simulink model "Symmetry_COPY"  (Simulink 8.1)
settings: Solver=ode23t  StartTime=0.0  StopTime=tfin  RelTol=1e-4
values from neighbouring files (symbols this model uses):
  amp_feedback_saturation = 400    [Symmetry_ini_COPY.m]
  Butterworth_filter_order = 8    [Sketch_controller_model_ini.m]    (also in Symmetry_ini.m; Symmetry_ini_COPY.m)
  C_Network = [0, 0, 0]    [Symmetry_ini.m]    (also in Symmetry_ini_COPY.m)
  Capacitive_Load_R_RC = [30e-3,  60e-3,  40e-3;                                1e-3, 5e-3, 3e-3]    [Symmetry_ini.m]    (also in Symmetry_ini_COPY.m = [60e-3,  120e-3,  80e-3;                                1e-3)
  Capacitive_Load_R_Switching_Sequence = Capacitive_Load_R_Switching_Sequence_'    [Symmetry_ini.m]    (also in Symmetry_ini_COPY.m = ones(3,tfin/Capacitive_Load_R_Switching_Speed(1))')
  Capacitive_Load_R_Switching_Speed = [0.01,0.01,0.01]    [Symmetry_ini.m]    (also in Symmetry_ini_COPY.m)
  Capacitive_Load_S_RC = [30e-3,  60e-3,  40e-3;                                1e-3, 5e-3, 3e-3]    [Symmetry_ini.m]    (also in Symmetry_ini_COPY.m = [60e-3,  120e-3,  80e-3;                                1e-3)
  Capacitive_Load_S_Switching_Sequence = Capacitive_Load_S_Switching_Sequence_'    [Symmetry_ini.m]    (also in Symmetry_ini_COPY.m = ones(3,tfin/Capacitive_Load_R_Switching_Speed(1))')
  Capacitive_Load_S_Switching_Speed = [0.01,0.01,0.01]    [Symmetry_ini.m]    (also in Symmetry_ini_COPY.m)
  Capacitive_Load_T_RC = [30e-3,  60e-3,  40e-3;                                1e-3, 5e-3, 3e-3]    [Symmetry_ini.m]    (also in Symmetry_ini_COPY.m = [60e-3,  120e-3,  80e-3;                                1e-3)
  Capacitive_Load_T_Switching_Sequence = Capacitive_Load_T_Switching_Sequence_'    [Symmetry_ini.m]    (also in Symmetry_ini_COPY.m = ones(3,tfin/Capacitive_Load_R_Switching_Speed(1))')
  Capacitive_Load_T_Switching_Speed = [0.01,0.01,0.01]    [Symmetry_ini.m]    (also in Symmetry_ini_COPY.m)
  i = str2num(answer{1})/sample    [Test_intersect.m]
  initial_value = [1,1,1,                  0,-2/3*pi,-4/3*pi]    [Symmetry_ini_COPY.m]
  L_Network = [3.185e-3, 3.185e-3, 3.185e-3, 3.185e-3]    [Symmetry_ini.m]    (also in Symmetry_ini_COPY.m)
  L_Source = [3.185e-3, 3.185e-3, 3.185e-3]    [Sketch_controller_model_ini.m]    (also in Symmetry_ini.m; Symmetry_ini_COPY.m)
  Load_R = [50,50,50]    [Symmetry_ini.m]    (also in Symmetry_ini_COPY.m)
  Load_RL = [35.35,   35.35,   35.35;                  0.1125,  0.1125,  0.1125]    [Symmetry_ini.m]    (also in Symmetry_ini_COPY.m)
  Load_Wire_Resistance = [0.1,0.2]    [Symmetry_ini.m]    (also in Symmetry_ini_COPY.m)
  P_gain = 0.01    [Symmetry_ini_COPY.m]
  phase_feedback_saturation = pi    (= 3.14159265359)    [Symmetry_ini_COPY.m]
  Phase_Source = [0,2/3*pi,4/3*pi]    [Sketch_controller_model_ini.m]    (also in Symmetry_REAL_TIME_ini.m = [0,-2/3*pi,-4/3*pi]; Symmetry_ini.m; Symmetry_ini_COPY.m = [0,-2/3*pi,-4/3*pi])
  R_Network = [0.4, 0.4, 0.4, 0.4]    [Symmetry_ini.m]    (also in Symmetry_ini_COPY.m)
  R_Source = [0.4, 0.4, 0.4]    [Sketch_controller_model_ini.m]    (also in Symmetry_ini.m; Symmetry_ini_COPY.m)
  sample = 10e-5    (= 0.0001)    [Inverter_ini.m]    (also in Sketch_controller_model_ini.m; Symmetry_REAL_TIME_ini.m; Symmetry_ini.m; Symmetry_ini_COPY.m)
  Source_Frequency = [50,50,50]    [Sketch_controller_model_ini.m]    (also in Symmetry_ini.m; Symmetry_ini_COPY.m)
  Start_Control = 0.1    [Symmetry_ini_COPY.m]
  step_size = [5,5,5,                  0.32,0.32,0.32]    [Symmetry_ini_COPY.m]
  Switch_Load_R = [1,1,1]    [Symmetry_ini.m]    (also in Symmetry_ini_COPY.m = [1,0,0])
  Switch_Load_RC = [1,1,1]    [Symmetry_ini.m]    (also in Symmetry_ini_COPY.m = [0,0,1])
  Switch_Load_RL = [1,1,1]    [Symmetry_ini.m]    (also in Symmetry_ini_COPY.m = [0,1,0])
  test_step = [1,1,1,                  0.08,0.08,0.08]    [Symmetry_ini_COPY.m]
  Urms_Source = [230,230,230]    [Sketch_controller_model_ini.m]    (also in Symmetry_REAL_TIME_ini.m; Symmetry_ini.m; Symmetry_ini_COPY.m)
libraries: powerlib x87, simulink x27, powerlib_extras x12, dspsigops x10, commsequence2 x6, dspxfrm3 x3, dsparch4 x3
(part 2 of 2)

== system Symmetry_COPY/Load System/Loads/Inductive_Loads_RST ==
  Breaker1 : powerlib/Elements/Breaker  BreakerResistance=0.01  InitialState=0  SnubberResistance=1e7  SnubberCapacitance=inf  SwitchingTimes="[ 1/60  5/60 ]"  External=on  Measurements=None  MoreParameters=off  NoBreakLoop=off
  Breaker13 : powerlib/Elements/Breaker  BreakerResistance=0.01  InitialState=0  SnubberResistance=1e7  SnubberCapacitance=inf  SwitchingTimes="[ 1/60  5/60 ]"  External=on  Measurements=None  MoreParameters=off  NoBreakLoop=off
  Breaker2 : powerlib/Elements/Breaker  BreakerResistance=0.01  InitialState=0  SnubberResistance=1e7  SnubberCapacitance=inf  SwitchingTimes="[ 1/60  5/60 ]"  External=on  Measurements=None  MoreParameters=off  NoBreakLoop=off
  Constant : Constant  Value=Switch_Load_RL(1)
  Constant1 : Constant  Value=Switch_Load_RL(2)
  Constant2 : Constant  Value=Switch_Load_RL(3)
  RL_load : powerlib/Elements/Series RLC Branch  LConnTagsString=__new0  RConnTagsString=__new0  BranchType=RL  Resistance=Load_RL(1,1)  Inductance=Load_RL(2,1)  SetiL0=off  InitialCurrent=0  Capacitance=1.0  Setx0=off  InitialVoltage=0  Measurements=None
  RL_load1 : powerlib/Elements/Series RLC Branch  LConnTagsString=__new0  RConnTagsString=__new0  BranchType=RL  Resistance=Load_RL(1,2)  Inductance=Load_RL(2,2)  SetiL0=off  InitialCurrent=0  Capacitance=1.0  Setx0=off  InitialVoltage=0  Measurements=None
  RL_load2 : powerlib/Elements/Series RLC Branch  LConnTagsString=__new0  RConnTagsString=__new0  BranchType=RL  Resistance=Load_RL(1,3)  Inductance=Load_RL(2,3)  SetiL0=off  InitialCurrent=0  Capacitance=1.0  Setx0=off  InitialVoltage=0  Measurements=None
  R : PMIOPort  Port=1  Side=Left
  S : PMIOPort  Port=2  Side=Left
  T : PMIOPort  Port=3  Side=Left
  N : PMIOPort  Port=4  Side=Right
  wires:
  Constant/1 -> Breaker13/1
  Constant1/1 -> Breaker1/1
  Constant2/1 -> Breaker2/1
  connections:
  RL_load/RConn1 -- RL_load1/RConn1 -- RL_load2/RConn1 -- N/RConn1
  R/RConn1 -- Breaker13/LConn1
  Breaker1/LConn1 -- S/RConn1
  Breaker2/LConn1 -- T/RConn1
  Breaker13/RConn1 -- RL_load/LConn1
  RL_load1/LConn1 -- Breaker1/RConn1
  RL_load2/LConn1 -- Breaker2/RConn1

== system Symmetry_COPY/Load System/Loads/Ohmic_Loads_RST ==
  Breaker1 : powerlib/Elements/Breaker  BreakerResistance=0.01  InitialState=0  SnubberResistance=1e7  SnubberCapacitance=inf  SwitchingTimes="[ 1/60  5/60 ]"  External=on  Measurements=None  MoreParameters=off  NoBreakLoop=off
  Breaker13 : powerlib/Elements/Breaker  BreakerResistance=0.01  InitialState=0  SnubberResistance=1e7  SnubberCapacitance=inf  SwitchingTimes="[ 1/60  5/60 ]"  External=on  Measurements=None  MoreParameters=off  NoBreakLoop=off
  Breaker2 : powerlib/Elements/Breaker  BreakerResistance=0.01  InitialState=0  SnubberResistance=1e7  SnubberCapacitance=inf  SwitchingTimes="[ 1/60  5/60 ]"  External=on  Measurements=None  MoreParameters=off  NoBreakLoop=off
  Constant : Constant  Value=Switch_Load_R(1)
  Constant1 : Constant  Value=Switch_Load_R(2)
  Constant2 : Constant  Value=Switch_Load_R(3)
  R_load : powerlib/Elements/Series RLC Branch  LConnTagsString=__new0  RConnTagsString=__new0  BranchType=R  Resistance=Load_R(1)  Inductance=0.003185  SetiL0=off  InitialCurrent=0  Capacitance=1.0  Setx0=off  InitialVoltage=0  Measurements=None
  R_load1 : powerlib/Elements/Series RLC Branch  LConnTagsString=__new0  RConnTagsString=__new0  BranchType=R  Resistance=Load_R(2)  Inductance=0.003185  SetiL0=off  InitialCurrent=0  Capacitance=1.0  Setx0=off  InitialVoltage=0  Measurements=None
  R_load2 : powerlib/Elements/Series RLC Branch  LConnTagsString=__new0  RConnTagsString=__new0  BranchType=R  Resistance=Load_R(3)  Inductance=0.003185  SetiL0=off  InitialCurrent=0  Capacitance=1.0  Setx0=off  InitialVoltage=0  Measurements=None
  R : PMIOPort  Port=1  Side=Left
  S : PMIOPort  Port=2  Side=Left
  T : PMIOPort  Port=3  Side=Left
  N : PMIOPort  Port=4  Side=Right
  wires:
  Constant/1 -> Breaker13/1
  Constant1/1 -> Breaker1/1
  Constant2/1 -> Breaker2/1
  connections:
  R_load/RConn1 -- R_load1/RConn1 -- R_load2/RConn1 -- N/RConn1
  Breaker13/LConn1 -- R/RConn1
  Breaker13/RConn1 -- R_load/LConn1
  Breaker1/LConn1 -- S/RConn1
  R_load1/LConn1 -- Breaker1/RConn1
  Breaker2/LConn1 -- T/RConn1
  R_load2/LConn1 -- Breaker2/RConn1

== system Symmetry_COPY/Load System/Log_Signals/3_Phase_P_Q ==
  U_RMS : Inport
  I_RMS : Inport  Port=2
  Demux1 : Demux  Outputs=3
  Demux3 : Demux  Outputs=3
  Mux4 : Mux  Inputs=3
  P Q in3 : powerlib_extras/Measurements/Active & Reactive Power  f1=Source_Frequency(1)
  P Q in4 : powerlib_extras/Measurements/Active & Reactive Power  f1=Source_Frequency(2)
  P Q in5 : powerlib_extras/Measurements/Active & Reactive Power  f1=Source_Frequency(3)
  P_Q_RMS : Outport
  wires:
  I_RMS/1 -> Demux1/1
  Demux1/3 -> P Q in5/2
  Demux1/2 -> P Q in4/2
  Demux1/1 -> P Q in3/2
  Demux3/3 -> P Q in5/1
  Demux3/2 -> P Q in4/1
  Demux3/1 -> P Q in3/1
  P Q in5/1 -> Mux4/3
  Mux4/1 -> P_Q_RMS/1
  U_RMS/1 -> Demux3/1
  P Q in4/1 -> Mux4/2
  P Q in3/1 -> Mux4/1

== system Symmetry_COPY/Load System/Log_Signals/3_Phase_RMS ==
  U_RST : Inport
  Demux5 : Demux  Outputs=3
  Mux2 : Mux  Inputs=3
  RMS1 : powerlib_extras/Measurements/RMS  f1=Source_Frequency(2)
  RMS2 : powerlib_extras/Measurements/RMS  f1=Source_Frequency(3)
  RMS6 : powerlib_extras/Measurements/RMS  f1=Source_Frequency(1)
  U_RMS : Outport
  wires:
  RMS2/1 -> Mux2/3
  Demux5/2 -> RMS1/1
  U_RST/1 -> Demux5/1
  Demux5/3 -> RMS2/1
  RMS6/1 -> Mux2/1
  Demux5/1 -> RMS6/1
  RMS1/1 -> Mux2/2
  Mux2/1 -> U_RMS/1

== system Symmetry_COPY/Load System/Log_Signals/3_Phase_RMS1 ==
  I_RST : Inport
  Demux5 : Demux  Outputs=3
  Mux2 : Mux  Inputs=3
  RMS1 : powerlib_extras/Measurements/RMS  f1=Source_Frequency(2)
  RMS2 : powerlib_extras/Measurements/RMS  f1=Source_Frequency(3)
  RMS6 : powerlib_extras/Measurements/RMS  f1=Source_Frequency(1)
  I_RMS : Outport
  wires:
  Demux5/3 -> RMS2/1
  Demux5/2 -> RMS1/1
  Demux5/1 -> RMS6/1
  Mux2/1 -> I_RMS/1
  RMS1/1 -> Mux2/2
  RMS6/1 -> Mux2/1
  I_RST/1 -> Demux5/1
  RMS2/1 -> Mux2/3

== system Symmetry_COPY/Load System/Log_Signals/3_Phase_THD ==
  U_RST : Inport
  Demux1 : Demux  Outputs=3
  Mux7 : Mux  Inputs=3
  THD1 : powerlib_extras/Measurements/Total Harmonic Distortion  f1=Source_Frequency(2)
  THD2 : powerlib_extras/Measurements/Total Harmonic Distortion  f1=Source_Frequency(3)
  THD3 : powerlib_extras/Measurements/Total Harmonic Distortion  f1=Source_Frequency(1)
  THD_RST : Outport
  wires:
  THD1/1 -> Mux7/2
  THD2/1 -> Mux7/3
  THD3/1 -> Mux7/1
  Demux1/3 -> THD2/1
  Mux7/1 -> THD_RST/1
  U_RST/1 -> Demux1/1
  Demux1/2 -> THD1/1
  Demux1/1 -> THD3/1

== system Symmetry_COPY/Load System/Loads/Capacitive_Loads_RST/Capacitive_Load_R ==
  Capacitive_Load_R_1 : Subsystem
  Capacitive_Load_R_2 : Subsystem
  Capacitive_Load_R_3 : Subsystem
  AC : PMIOPort  Port=1  Side=Left
  N : PMIOPort  Port=2  Side=Left
  connections:
  N/RConn1 -- Capacitive_Load_R_3/LConn2 -- Capacitive_Load_R_2/LConn2 -- Capacitive_Load_R_1/RConn2
  Capacitive_Load_R_2/LConn1 -- Capacitive_Load_R_1/RConn1 -- Capacitive_Load_R_3/LConn1 -- AC/RConn1

== system Symmetry_COPY/Load System/Loads/Capacitive_Loads_RST/Capacitive_Load_S ==
  Capacitive_Load_S_1 : Subsystem
  Capacitive_Load_S_2 : Subsystem
  Capacitive_Load_S_3 : Subsystem
  AC : PMIOPort  Port=1  Side=Left
  N : PMIOPort  Port=2  Side=Left
  connections:
  AC/RConn1 -- Capacitive_Load_S_3/LConn1 -- Capacitive_Load_S_1/RConn1 -- Capacitive_Load_S_2/LConn1
  Capacitive_Load_S_1/RConn2 -- Capacitive_Load_S_2/LConn2 -- Capacitive_Load_S_3/LConn2 -- N/RConn1

== system Symmetry_COPY/Load System/Loads/Capacitive_Loads_RST/Capacitive_Load_T ==
  Capacitive_Load_R_1 : Subsystem
  Capacitive_Load_R_2 : Subsystem
  Capacitive_Load_R_3 : Subsystem
  AC : PMIOPort  Port=1  Side=Left
  N : PMIOPort  Port=2  Side=Left
  connections:
  N/RConn1 -- Capacitive_Load_R_3/LConn2 -- Capacitive_Load_R_2/LConn2 -- Capacitive_Load_R_1/RConn2
  Capacitive_Load_R_2/LConn1 -- Capacitive_Load_R_1/RConn1 -- Capacitive_Load_R_3/LConn1 -- AC/RConn1

== system Symmetry_COPY/Load System/Loads/Capacitive_Loads_RST/Capacitive_Load_R/Capacitive_Load_R_1 ==
  Breaker5 : powerlib/Elements/Breaker  BreakerResistance=0.01  InitialState=0  SnubberResistance=1e7  SnubberCapacitance=inf  SwitchingTimes="[ 1/60  5/60 ]"  External=on  Measurements=None  MoreParameters=off  NoBreakLoop=off
  Ron3 : simulink/Sources/Repeating Sequence Stair  OutValues=Capacitive_Load_R_Switching_Sequence(:,1)  tsamp=Capacitive_Load_R_Switching_Speed(1)  OutMin=[]  OutMax=[]  OutDataTypeStr=float('double')  OutputDataTypeScalingMode=Specify via dialog  OutDataType=float('double')  ConRadixGroup=Best Precision: Vector-wise  OutScaling=2^-12
  Series RLC Branch : powerlib/Elements/Series RLC Branch  LConnTagsString=__new0  RConnTagsString=__new0  BranchType=RC  Resistance=Capacitive_Load_R_RC(1,1)  Inductance=1e-3  SetiL0=off  InitialCurrent=0  Capacitance=Capacitive_Load_R_RC(2,1)  Setx0=off  InitialVoltage=0  Measurements=None
  Universal Bridge : powerlib/Power Electronics/Universal Bridge  Arms=2  SnubberResistance=1e5  SnubberCapacitance=inf  Device=Diodes  Ron=1e-3  Lon=0  ForwardVoltages="[  0  0  ]"  ForwardVoltage=0.8  GTOparameters=[ 10e-6 , 20e-6 ]  IGBTparameters=[ 1e-6 , 2e-6 ]  Measurements=None  Measurements_2=None  converterType=Rectifier
  AC : PMIOPort  Port=1  Side=Right
  N : PMIOPort  Port=2  Side=Right
  wires:
  Ron3/1 -> Breaker5/1
  connections:
  Universal Bridge/LConn2 -- N/RConn1
  Breaker5/RConn1 -- Universal Bridge/LConn1
  AC/RConn1 -- Breaker5/LConn1
  Universal Bridge/RConn1 -- Series RLC Branch/LConn1
  Universal Bridge/RConn2 -- Series RLC Branch/RConn1

== system Symmetry_COPY/Load System/Loads/Capacitive_Loads_RST/Capacitive_Load_R/Capacitive_Load_R_2 ==
  Breaker2 : powerlib/Elements/Breaker  BreakerResistance=0.01  InitialState=0  SnubberResistance=1e7  SnubberCapacitance=inf  SwitchingTimes="[ 1/60  5/60 ]"  External=on  Measurements=None  MoreParameters=off  NoBreakLoop=off
  Ron1 : simulink/Sources/Repeating Sequence Stair  OutValues=Capacitive_Load_R_Switching_Sequence(:,2)  tsamp=Capacitive_Load_R_Switching_Speed(2)  OutMin=[]  OutMax=[]  OutDataTypeStr=float('double')  OutputDataTypeScalingMode=Specify via dialog  OutDataType=float('double')  ConRadixGroup=Best Precision: Vector-wise  OutScaling=2^-12
  Series RLC Branch : powerlib/Elements/Series RLC Branch  LConnTagsString=__new0  RConnTagsString=__new0  BranchType=RC  Resistance=Capacitive_Load_R_RC(1,2)  Inductance=1e-3  SetiL0=off  InitialCurrent=0  Capacitance=Capacitive_Load_R_RC(2,2)  Setx0=off  InitialVoltage=0  Measurements=None
  Universal Bridge1 : powerlib/Power Electronics/Universal Bridge  Arms=2  SnubberResistance=1e5  SnubberCapacitance=inf  Device=Diodes  Ron=1e-3  Lon=0  ForwardVoltages="[  0  0  ]"  ForwardVoltage=0.8  GTOparameters=[ 10e-6 , 20e-6 ]  IGBTparameters=[ 1e-6 , 2e-6 ]  Measurements=None  Measurements_2=None  converterType=Rectifier
  AC : PMIOPort  Port=1  Side=Left
  N : PMIOPort  Port=2  Side=Left
  wires:
  Ron1/1 -> Breaker2/1
  connections:
  Universal Bridge1/LConn2 -- N/RConn1
  Breaker2/RConn1 -- Universal Bridge1/LConn1
  AC/RConn1 -- Breaker2/LConn1
  Series RLC Branch/LConn1 -- Universal Bridge1/RConn1
  Series RLC Branch/RConn1 -- Universal Bridge1/RConn2

== system Symmetry_COPY/Load System/Loads/Capacitive_Loads_RST/Capacitive_Load_R/Capacitive_Load_R_3 ==
  Breaker3 : powerlib/Elements/Breaker  BreakerResistance=0.01  InitialState=0  SnubberResistance=1e7  SnubberCapacitance=inf  SwitchingTimes="[ 1/60  5/60 ]"  External=on  Measurements=None  MoreParameters=off  NoBreakLoop=off
  Ron4 : simulink/Sources/Repeating Sequence Stair  OutValues=Capacitive_Load_R_Switching_Sequence(:,3)  tsamp=Capacitive_Load_R_Switching_Speed(3)  OutMin=[]  OutMax=[]  OutDataTypeStr=float('double')  OutputDataTypeScalingMode=Specify via dialog  OutDataType=float('double')  ConRadixGroup=Best Precision: Vector-wise  OutScaling=2^-12
  Series RLC Branch : powerlib/Elements/Series RLC Branch  LConnTagsString=__new0  RConnTagsString=__new0  BranchType=RC  Resistance=Capacitive_Load_R_RC(1,3)  Inductance=1e-3  SetiL0=off  InitialCurrent=0  Capacitance=Capacitive_Load_R_RC(2,3)  Setx0=off  InitialVoltage=0  Measurements=None
  Universal Bridge2 : powerlib/Power Electronics/Universal Bridge  Arms=2  SnubberResistance=1e5  SnubberCapacitance=inf  Device=Diodes  Ron=1e-3  Lon=0  ForwardVoltages="[  0  0  ]"  ForwardVoltage=0.8  GTOparameters=[ 10e-6 , 20e-6 ]  IGBTparameters=[ 1e-6 , 2e-6 ]  Measurements=None  Measurements_2=None  converterType=Rectifier
  AC : PMIOPort  Port=1  Side=Left
  "N " : PMIOPort  Port=2  Side=Left
  wires:
  Ron4/1 -> Breaker3/1
  connections:
  Breaker3/RConn1 -- Universal Bridge2/LConn1
  Universal Bridge2/LConn2 -- "N "/RConn1
  AC/RConn1 -- Breaker3/LConn1
  Series RLC Branch/LConn1 -- Universal Bridge2/RConn1
  Series RLC Branch/RConn1 -- Universal Bridge2/RConn2

== system Symmetry_COPY/Load System/Loads/Capacitive_Loads_RST/Capacitive_Load_S/Capacitive_Load_S_1 ==
  Breaker5 : powerlib/Elements/Breaker  BreakerResistance=0.01  InitialState=0  SnubberResistance=1e7  SnubberCapacitance=inf  SwitchingTimes="[ 1/60  5/60 ]"  External=on  Measurements=None  MoreParameters=off  NoBreakLoop=off
  Ron3 : simulink/Sources/Repeating Sequence Stair  OutValues=Capacitive_Load_S_Switching_Sequence(:,1)  tsamp=Capacitive_Load_S_Switching_Speed(1)  OutMin=[]  OutMax=[]  OutDataTypeStr=float('double')  OutputDataTypeScalingMode=Specify via dialog  OutDataType=float('double')  ConRadixGroup=Best Precision: Vector-wise  OutScaling=2^-12
  Series RLC Branch : powerlib/Elements/Series RLC Branch  LConnTagsString=__new0  RConnTagsString=__new0  BranchType=RC  Resistance=Capacitive_Load_S_RC(1,1)  Inductance=1e-3  SetiL0=off  InitialCurrent=0  Capacitance=Capacitive_Load_S_RC(2,1)  Setx0=off  InitialVoltage=0  Measurements=None
  Universal Bridge : powerlib/Power Electronics/Universal Bridge  Arms=2  SnubberResistance=1e5  SnubberCapacitance=inf  Device=Diodes  Ron=1e-3  Lon=0  ForwardVoltages="[  0  0  ]"  ForwardVoltage=0.8  GTOparameters=[ 10e-6 , 20e-6 ]  IGBTparameters=[ 1e-6 , 2e-6 ]  Measurements=None  Measurements_2=None  converterType=Rectifier
  AC : PMIOPort  Port=1  Side=Right
  N : PMIOPort  Port=2  Side=Right
  wires:
  Ron3/1 -> Breaker5/1
  connections:
  AC/RConn1 -- Breaker5/LConn1
  Breaker5/RConn1 -- Universal Bridge/LConn1
  Universal Bridge/LConn2 -- N/RConn1
  Series RLC Branch/LConn1 -- Universal Bridge/RConn1
  Series RLC Branch/RConn1 -- Universal Bridge/RConn2

== system Symmetry_COPY/Load System/Loads/Capacitive_Loads_RST/Capacitive_Load_S/Capacitive_Load_S_2 ==
  Breaker2 : powerlib/Elements/Breaker  BreakerResistance=0.01  InitialState=0  SnubberResistance=1e7  SnubberCapacitance=inf  SwitchingTimes="[ 1/60  5/60 ]"  External=on  Measurements=None  MoreParameters=off  NoBreakLoop=off
  Ron1 : simulink/Sources/Repeating Sequence Stair  OutValues=Capacitive_Load_S_Switching_Sequence(:,2)  tsamp=Capacitive_Load_S_Switching_Speed(2)  OutMin=[]  OutMax=[]  OutDataTypeStr=float('double')  OutputDataTypeScalingMode=Specify via dialog  OutDataType=float('double')  ConRadixGroup=Best Precision: Vector-wise  OutScaling=2^-12
  Series RLC Branch : powerlib/Elements/Series RLC Branch  LConnTagsString=__new0  RConnTagsString=__new0  BranchType=RC  Resistance=Capacitive_Load_S_RC(1,2)  Inductance=1e-3  SetiL0=off  InitialCurrent=0  Capacitance=Capacitive_Load_S_RC(2,2)  Setx0=off  InitialVoltage=0  Measurements=None
  Universal Bridge1 : powerlib/Power Electronics/Universal Bridge  Arms=2  SnubberResistance=1e5  SnubberCapacitance=inf  Device=Diodes  Ron=1e-3  Lon=0  ForwardVoltages="[  0  0  ]"  ForwardVoltage=0.8  GTOparameters=[ 10e-6 , 20e-6 ]  IGBTparameters=[ 1e-6 , 2e-6 ]  Measurements=None  Measurements_2=None  converterType=Rectifier
  AC : PMIOPort  Port=1  Side=Left
  N : PMIOPort  Port=2  Side=Left
  wires:
  Ron1/1 -> Breaker2/1
  connections:
  AC/RConn1 -- Breaker2/LConn1
  Breaker2/RConn1 -- Universal Bridge1/LConn1
  Universal Bridge1/LConn2 -- N/RConn1
  Series RLC Branch/LConn1 -- Universal Bridge1/RConn1
  Series RLC Branch/RConn1 -- Universal Bridge1/RConn2

== system Symmetry_COPY/Load System/Loads/Capacitive_Loads_RST/Capacitive_Load_S/Capacitive_Load_S_3 ==
  Breaker3 : powerlib/Elements/Breaker  BreakerResistance=0.01  InitialState=0  SnubberResistance=1e7  SnubberCapacitance=inf  SwitchingTimes="[ 1/60  5/60 ]"  External=on  Measurements=None  MoreParameters=off  NoBreakLoop=off
  Ron4 : simulink/Sources/Repeating Sequence Stair  OutValues=Capacitive_Load_S_Switching_Sequence(:,3)  tsamp=Capacitive_Load_S_Switching_Speed(3)  OutMin=[]  OutMax=[]  OutDataTypeStr=float('double')  OutputDataTypeScalingMode=Specify via dialog  OutDataType=float('double')  ConRadixGroup=Best Precision: Vector-wise  OutScaling=2^-12
  Series RLC Branch : powerlib/Elements/Series RLC Branch  LConnTagsString=__new0  RConnTagsString=__new0  BranchType=RC  Resistance=Capacitive_Load_S_RC(1,3)  Inductance=1e-3  SetiL0=off  InitialCurrent=0  Capacitance=Capacitive_Load_S_RC(2,3)  Setx0=off  InitialVoltage=0  Measurements=None
  Universal Bridge2 : powerlib/Power Electronics/Universal Bridge  Arms=2  SnubberResistance=1e5  SnubberCapacitance=inf  Device=Diodes  Ron=1e-3  Lon=0  ForwardVoltages="[  0  0  ]"  ForwardVoltage=0.8  GTOparameters=[ 10e-6 , 20e-6 ]  IGBTparameters=[ 1e-6 , 2e-6 ]  Measurements=None  Measurements_2=None  converterType=Rectifier
  AC : PMIOPort  Port=1  Side=Left
  "N " : PMIOPort  Port=2  Side=Left
  wires:
  Ron4/1 -> Breaker3/1
  connections:
  AC/RConn1 -- Breaker3/LConn1
  Universal Bridge2/LConn2 -- "N "/RConn1
  Breaker3/RConn1 -- Universal Bridge2/LConn1
  Series RLC Branch/LConn1 -- Universal Bridge2/RConn1
  Series RLC Branch/RConn1 -- Universal Bridge2/RConn2

== system Symmetry_COPY/Load System/Loads/Capacitive_Loads_RST/Capacitive_Load_T/Capacitive_Load_R_1 ==
  Breaker5 : powerlib/Elements/Breaker  BreakerResistance=0.01  InitialState=0  SnubberResistance=1e7  SnubberCapacitance=inf  SwitchingTimes="[ 1/60  5/60 ]"  External=on  Measurements=None  MoreParameters=off  NoBreakLoop=off
  Ron3 : simulink/Sources/Repeating Sequence Stair  OutValues=Capacitive_Load_T_Switching_Sequence(:,1)  tsamp=Capacitive_Load_T_Switching_Speed(1)  OutMin=[]  OutMax=[]  OutDataTypeStr=float('double')  OutputDataTypeScalingMode=Specify via dialog  OutDataType=float('double')  ConRadixGroup=Best Precision: Vector-wise  OutScaling=2^-12
  Series RLC Branch : powerlib/Elements/Series RLC Branch  LConnTagsString=__new0  RConnTagsString=__new0  BranchType=RC  Resistance=Capacitive_Load_T_RC(1,1)  Inductance=1e-3  SetiL0=off  InitialCurrent=0  Capacitance=Capacitive_Load_T_RC(2,1)  Setx0=off  InitialVoltage=0  Measurements=None
  Universal Bridge : powerlib/Power Electronics/Universal Bridge  Arms=2  SnubberResistance=1e5  SnubberCapacitance=inf  Device=Diodes  Ron=1e-3  Lon=0  ForwardVoltages="[  0  0  ]"  ForwardVoltage=0.8  GTOparameters=[ 10e-6 , 20e-6 ]  IGBTparameters=[ 1e-6 , 2e-6 ]  Measurements=None  Measurements_2=None  converterType=Rectifier
  AC : PMIOPort  Port=1  Side=Right
  N : PMIOPort  Port=2  Side=Right
  wires:
  Ron3/1 -> Breaker5/1
  connections:
  Universal Bridge/LConn2 -- N/RConn1
  Breaker5/RConn1 -- Universal Bridge/LConn1
  AC/RConn1 -- Breaker5/LConn1
  Series RLC Branch/RConn1 -- Universal Bridge/RConn2
  Series RLC Branch/LConn1 -- Universal Bridge/RConn1

== system Symmetry_COPY/Load System/Loads/Capacitive_Loads_RST/Capacitive_Load_T/Capacitive_Load_R_2 ==
  Breaker2 : powerlib/Elements/Breaker  BreakerResistance=0.01  InitialState=0  SnubberResistance=1e7  SnubberCapacitance=inf  SwitchingTimes="[ 1/60  5/60 ]"  External=on  Measurements=None  MoreParameters=off  NoBreakLoop=off
  Ron1 : simulink/Sources/Repeating Sequence Stair  OutValues=Capacitive_Load_T_Switching_Sequence(:,2)  tsamp=Capacitive_Load_T_Switching_Speed(2)  OutMin=[]  OutMax=[]  OutDataTypeStr=float('double')  OutputDataTypeScalingMode=Specify via dialog  OutDataType=float('double')  ConRadixGroup=Best Precision: Vector-wise  OutScaling=2^-12
  Series RLC Branch : powerlib/Elements/Series RLC Branch  LConnTagsString=__new0  RConnTagsString=__new0  BranchType=RC  Resistance=Capacitive_Load_T_RC(1,2)  Inductance=1e-3  SetiL0=off  InitialCurrent=0  Capacitance=Capacitive_Load_T_RC(2,2)  Setx0=off  InitialVoltage=0  Measurements=None
  Universal Bridge1 : powerlib/Power Electronics/Universal Bridge  Arms=2  SnubberResistance=1e5  SnubberCapacitance=inf  Device=Diodes  Ron=1e-3  Lon=0  ForwardVoltages="[  0  0  ]"  ForwardVoltage=0.8  GTOparameters=[ 10e-6 , 20e-6 ]  IGBTparameters=[ 1e-6 , 2e-6 ]  Measurements=None  Measurements_2=None  converterType=Rectifier
  AC : PMIOPort  Port=1  Side=Left
  N : PMIOPort  Port=2  Side=Left
  wires:
  Ron1/1 -> Breaker2/1
  connections:
  Universal Bridge1/LConn2 -- N/RConn1
  Breaker2/RConn1 -- Universal Bridge1/LConn1
  AC/RConn1 -- Breaker2/LConn1
  Series RLC Branch/RConn1 -- Universal Bridge1/RConn2
  Series RLC Branch/LConn1 -- Universal Bridge1/RConn1

== system Symmetry_COPY/Load System/Loads/Capacitive_Loads_RST/Capacitive_Load_T/Capacitive_Load_R_3 ==
  Breaker3 : powerlib/Elements/Breaker  BreakerResistance=0.01  InitialState=0  SnubberResistance=1e7  SnubberCapacitance=inf  SwitchingTimes="[ 1/60  5/60 ]"  External=on  Measurements=None  MoreParameters=off  NoBreakLoop=off
  Ron4 : simulink/Sources/Repeating Sequence Stair  OutValues=Capacitive_Load_T_Switching_Sequence(:,3)  tsamp=Capacitive_Load_T_Switching_Speed(3)  OutMin=[]  OutMax=[]  OutDataTypeStr=float('double')  OutputDataTypeScalingMode=Specify via dialog  OutDataType=float('double')  ConRadixGroup=Best Precision: Vector-wise  OutScaling=2^-12
  Series RLC Branch : powerlib/Elements/Series RLC Branch  LConnTagsString=__new0  RConnTagsString=__new0  BranchType=RC  Resistance=Capacitive_Load_T_RC(1,3)  Inductance=1e-3  SetiL0=off  InitialCurrent=0  Capacitance=Capacitive_Load_T_RC(2,3)  Setx0=off  InitialVoltage=0  Measurements=None
  Universal Bridge2 : powerlib/Power Electronics/Universal Bridge  Arms=2  SnubberResistance=1e5  SnubberCapacitance=inf  Device=Diodes  Ron=1e-3  Lon=0  ForwardVoltages="[  0  0  ]"  ForwardVoltage=0.8  GTOparameters=[ 10e-6 , 20e-6 ]  IGBTparameters=[ 1e-6 , 2e-6 ]  Measurements=None  Measurements_2=None  converterType=Rectifier
  AC : PMIOPort  Port=1  Side=Left
  "N " : PMIOPort  Port=2  Side=Left
  wires:
  Ron4/1 -> Breaker3/1
  connections:
  Breaker3/RConn1 -- Universal Bridge2/LConn1
  Universal Bridge2/LConn2 -- "N "/RConn1
  AC/RConn1 -- Breaker3/LConn1
  Series RLC Branch/RConn1 -- Universal Bridge2/RConn2
  Series RLC Branch/LConn1 -- Universal Bridge2/RConn1

== matlab function Calculate_Norms/Mearusement_calc/regular norm ==
  data: amplitude_R input double; REG_norm output double; amplitude_S input double; amplitude_T input double; phase_R input double; phase_S input double; phase_T input double
function REG_norm = fcn(amplitude_R,amplitude_S,amplitude_T,phase_R,phase_S,phase_T)
%#codegen

 A=(1/3)*[1,                1,                  1;...
          1,      exp(1i*120/360*2*pi),        exp(1i*240/360*2*pi);...
          1,      exp(1i*240/360*2*pi),       exp(1i*120/360*2*pi)];
   
   V_real=complex([0,0,0]');
   V_012=complex([0,0,0]');
   V_real(1)=amplitude_R.*exp(1i*phase_R);
   V_real(2)=amplitude_S.*exp(1i*phase_S);
   V_real(3)=amplitude_T.*exp(1i*phase_T); 
   V_012=A*V_real;
   REG_norm=(abs(V_012(3))/abs(V_012(2)))*100;

== matlab function Calculate_Norms/Mearusement_calc/vectorial norm ==
  data: amplitude_R input double; VEC_norm output double; amplitude_S input double; amplitude_T input double; phase_R input double; phase_S input double; phase_T input double
function VEC_norm = fcn(amplitude_R,amplitude_S,amplitude_T,phase_R,phase_S,phase_T)
%#codegen

  
   N=complex(0);
   V_real=complex([0,0,0]');
   V_012=complex([0,0,0]');
   V_real(1)=amplitude_R.*exp(1i*phase_R);
   V_real(2)=amplitude_S.*exp(1i*phase_S);
   V_real(3)=amplitude_T.*exp(1i*phase_T); 

   R_error=230*exp(1j*-0/360*2*pi)  -V_real(1);
   S_error=230*exp(1j*-120/360*2*pi)-V_real(2);
   T_error=230*exp(1j*-240/360*2*pi)-V_real(3);
   N=R_error*S_error+R_error*T_error+S_error*T_error;
   VEC_norm=abs(N);

== matlab function Calculate_Norms/Mearusement_calc/geometrial norm1 ==
  data: amplitude_R input double; GEO_norm output double; amplitude_S input double; amplitude_T input double; phase_R input double; phase_S input double; phase_T input double
function GEO_norm = fcn(amplitude_R,amplitude_S,amplitude_T,phase_R,phase_S,phase_T)
%#codegen

x1=[0,0,0,0];
y1=[0,0,0,0];
x2=[0,0,0,0];
y2=[0,0,0,0];

GEO_norm=0;

coder.extrinsic('geometry_solver')

        %% Ideal parameters
        Amplitude_1=[325.3,325.3,325.3];                     %[V]
        Phase_1=[-1.5855,2.6033,0.5089];
        %Phase_1=[0,-2/3*pi,-4/3*pi];                     %[rad]
      
        %% Real parameters
        Amplitude_2=[amplitude_R,amplitude_S,amplitude_T];
        Phase_2=[phase_R,phase_S,phase_T];
        %Extension of the vectors with the first element to get closed triangles on
        %plots and for use as polygons
        Amplitude_1_ex=[Amplitude_1 Amplitude_1(1)];
        Phase_1_ex=[Phase_1 Phase_1(1)];
        Amplitude_2_ex=[Amplitude_2 Amplitude_2(1)];
        Phase_2_ex=[Phase_2 Phase_2(1)];
        
        GEO_norm=geometry_solver(Amplitude_1_ex, Phase_1_ex, Amplitude_2_ex, Phase_2_ex);

== matlab function Control Current/MATLAB Function ==
  data: amp input double; CC output double; phase input double; t input double
function CC = fcn(amp,phase,t)
%#codegen


CC_mtx=[amp(1),50,phase(1),0;...
        amp(2),50,phase(2),0;...
        amp(3),50,phase(3),0];
% T=1;
% CC=[(CC_mtx(1,1)*sin(2*pi*CC_mtx(1,2)*t+CC_mtx(1,3))+CC_mtx(1,4)).*(1-exp(-t/T)),...
%     (CC_mtx(2,1)*sin(2*pi*CC_mtx(2,2)*t+CC_mtx(2,3))+CC_mtx(2,4)).*(1-exp(-t/T)),...
%     (CC_mtx(3,1)*sin(2*pi*CC_mtx(3,2)*t+CC_mtx(3,3))+CC_mtx(3,4)).*(1-exp(-t/T))]';

CC=[(CC_mtx(1,1)*sin(2*pi*CC_mtx(1,2)*t+CC_mtx(1,3))+CC_mtx(1,4)),...
    (CC_mtx(2,1)*sin(2*pi*CC_mtx(2,2)*t+CC_mtx(2,3))+CC_mtx(2,4)),...
    (CC_mtx(3,1)*sin(2*pi*CC_mtx(3,2)*t+CC_mtx(3,3))+CC_mtx(3,4))]';
